simulink model "modelo_lqr_gab"  (R2023a)
settings: Solver=VariableStepAuto  StartTime=0.0  StopTime=10.0  RelTol=1e-3
values from neighbouring files (symbols this model uses):
  Ard = [Ar(1,1) Ar(1,3:end) ... (first row only)    [Modelo_mono.m]    (also in workspace.mat = [0 0 -31.2551437046 31.2551437046 0 0 0 0 0 0 -92.3888975157)
  Brd = [Br(1,:) ... (first row only)    [Modelo_mono.m]    (also in workspace.mat = [0  0; 0  0; 50297.8358889  0; -78.116759971  0; 0  238.3657)
  Crd = [1 0 0 0 0 0 0 1 0 0 0 0 ... (36 elements, 6x6)]    [workspace.mat]
  K = lqr(Ard,Brd,Qc,Rc)    [Modelo_mono.m]    (also in cascatinha_v3.m = [tprK,0; workspace.mat = [-891.058429104  -1.00065730536e-12  -0.217264538579  -159.5)
  v_ic = [0;0;0;0]    [Modelo_mono.m]    (also in workspace.mat = [0 0 0 0])
  x_ic = [0;5*pi/180;0;-5*pi/180]    [Modelo_mono.m]    (also in workspace.mat = [0 0.0872664625997 0 -0.0872664625997])
settings Model: Creator=gabri  LastModifiedBy=pinki
settings OptimizationCC: ReuseModelBlockBuffer=off

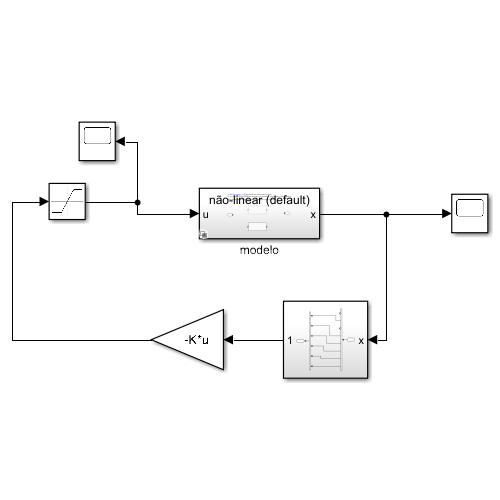
[thumbnail: Simulink's stored preview of the top-level diagram]
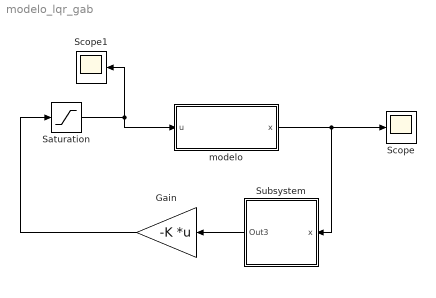
== system modelo_lqr_gab ==
  Gain : Gain  Gain=-K  Multiplication=Matrix(K*u)
  Saturation : Saturate  UpperLimit=1  LowerLimit=-1
  Scope : Scope
  Scope1 : Scope
  Subsystem : Subsystem
  modelo : Subsystem  Variant=on  VariantControlMode=label  LabelModeActiveChoice=(default)
  wires:
  Gain/1 -> Saturation/1
  Subsystem/1(Out3) -> Gain/1
  modelo/1(x) -> Scope/1, Subsystem/1(x)
  Saturation/1 -> modelo/1(u), Scope1/1

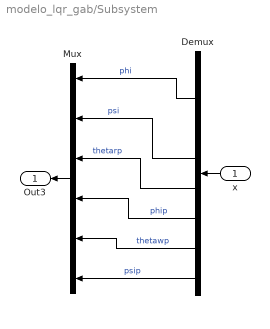
== system modelo_lqr_gab/Subsystem ==
  x : Inport
  Demux : Demux  Outputs=8
  Mux : Mux  Inputs=6
  Out3 : Outport
  wires:
  Demux/2 -> Mux/1  "phi"
  Demux/4 -> Mux/2  "psi"
  Demux/8 -> Mux/6  "psip"
  Demux/5 -> Mux/3  "thetarp"
  Demux/7 -> Mux/5  "thetawp"
  Demux/6 -> Mux/4  "phip"
  Mux/1 -> Out3/1
  x/1 -> Demux/1

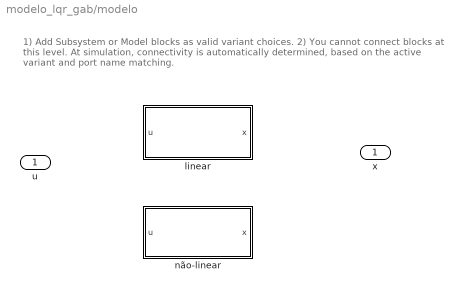
== system modelo_lqr_gab/modelo ==
  note: 1) Add Subsystem or Model blocks as valid variant choices.
      | 2) You cannot connect blocks at this level. At simulation, connectivity is automatically
      | determined, based on the active variant and port name matching.
  u : Inport
  linear : Subsystem  VariantControl=false
  não-linear : Subsystem  VariantControl=(default)
  x : Outport

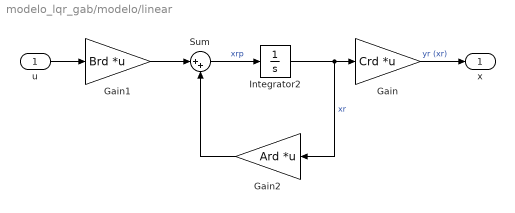
== system modelo_lqr_gab/modelo/linear ==
  u : Inport
  Gain : Gain  Gain=Crd  Multiplication=Matrix(K*u) (u vector)
  Gain1 : Gain  Gain=Brd  Multiplication=Matrix(K*u) (u vector)
  Gain2 : Gain  Gain=Ard  Multiplication=Matrix(K*u) (u vector)
  Integrator2 : Integrator  InitialCondition=x_ic
  Sum : Sum  Inputs=|++
  x : Outport
  wires:
  Gain2/1 -> Sum/2
  Gain1/1 -> Sum/1
  Integrator2/1 -> Gain2/1, Gain/1  "xr"
  u/1 -> Gain1/1
  Gain/1 -> x/1  "yr (xr)"
  Sum/1 -> Integrator2/1  "xrp"

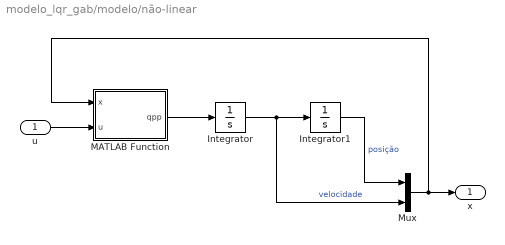
== system modelo_lqr_gab/modelo/não-linear ==
  u : Inport
  Integrator : Integrator  InitialCondition=v_ic
  Integrator1 : Integrator  InitialCondition=x_ic
  MATLAB Function : MATLAB Function  TreatAsAtomicUnit=on
  Mux : Mux  Inputs=2
  x : Outport
  wires:
  Integrator/1 -> Mux/2, Integrator1/1  "velocidade"
  MATLAB Function/1(qpp) -> Integrator/1
  u/1 -> MATLAB Function/2(u)
  Mux/1 -> MATLAB Function/1(x), x/1
  Integrator1/1 -> Mux/1  "posição"

== matlab function modelo_lqr_gab/modelo/não-linear/MATLAB Function ==
  data: x input; u input; qpp output
function qpp = fcn(x,u)

M = function_M(x(4));
V = function_V(x(6),x(4),x(8),x(5),x(7));
G = function_G(x(2),x(4));
P = function_P();

qpp = M^-1*(-V-G+P*u);
